simulink model "ModeleVehicule_2_0"  (R2018a)
settings: Solver=VariableStepAuto  StartTime=0.0  StopTime=3600  RelTol=1e-3
libraries: VehiculeHypothese x1, ForcesHypothese x1, ConducteurHypothese x1
settings Model: Creator=Thomas  LastModifiedBy=thomas.moser

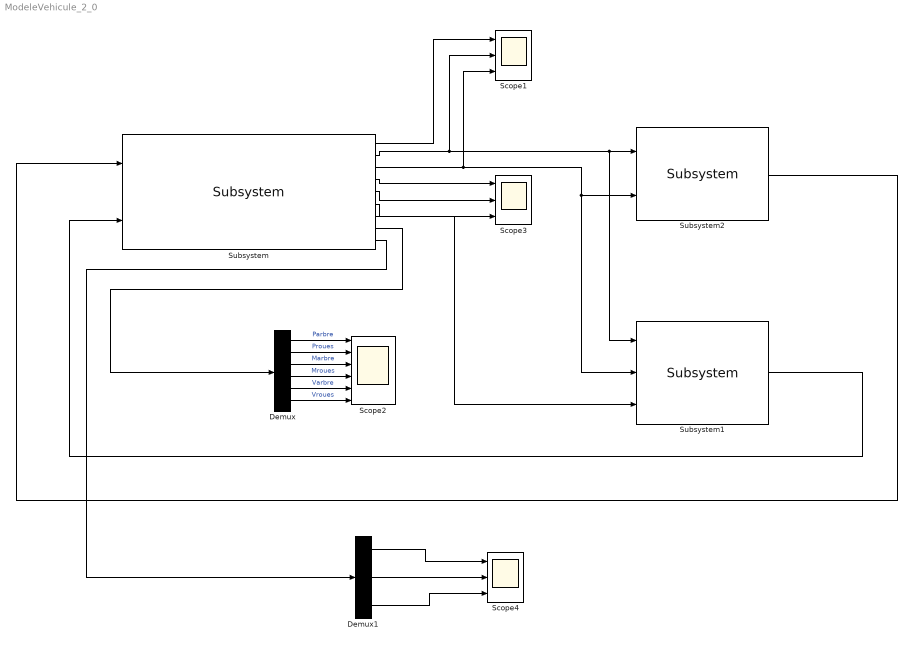
== system ModeleVehicule_2_0 ==
  Demux : Demux  Outputs=6
  Demux1 : Demux  Outputs=3
  Scope1 : Scope  NumInputPorts=3
  Scope2 : Scope  NumInputPorts=6
  Scope3 : Scope  NumInputPorts=3
  Scope4 : Scope  NumInputPorts=3
  Subsystem : VehiculeHypothese/Subsystem  m=2250  mp=80  rr=0.33  s=1  cx=0.5  crr=0.015  mlimit=660  alimit=3  r=9.73  nr=0.9  nm=0.89  nc=0.89  cb=98
      link override 1-D Lookup Table1: BreakpointsForDimension1=vitesseCouple  Table=seuilCoupleMax
      link override Saturation1: UpperLimit=mlimit*r*nr  LowerLimit=-mlimit*r*nr
  Subsystem1 : ForcesHypothese/Subsystem  rho=1.225  g=9.81
      link override 1-D Lookup Table2: BreakpointsForDimension1=c_dist_int(1:1:length(vlim)-1)  Table=alpha_int
  Subsystem2 : ConducteurHypothese/Subsystem  SystemSampleTime=-1
  wires:
  Subsystem/2 -> Subsystem2/1, Subsystem1/1, Scope1/2
  Subsystem/3 -> Subsystem1/2, Subsystem2/2, Scope1/3
  Subsystem1/1 -> Subsystem/2
  Subsystem/6 -> Scope3/3
  Subsystem/5 -> Scope3/2
  Subsystem/4 -> Scope3/1
  Subsystem/7 -> Subsystem1/3
  Subsystem/1 -> Scope1/1
  Subsystem/8 -> Demux/1
  Demux/1 -> Scope2/1  "Parbre"
  Demux/2 -> Scope2/2  "Proues"
  Demux/3 -> Scope2/3  "Marbre"
  Demux/4 -> Scope2/4  "Mroues"
  Demux/5 -> Scope2/5  "Varbre"
  Demux/6 -> Scope2/6  "Vroues"
  Subsystem2/1 -> Subsystem/1
  Subsystem/9 -> Demux1/1
  Demux1/1 -> Scope4/1
  Demux1/2 -> Scope4/2
  Demux1/3 -> Scope4/3
